simulink model "Synapse"  (Simulink 8.4)
settings: Solver=ode45  StartTime=0.0  StopTime=0.5  RelTol=1e-3
libraries: NeuroModelerLibrary x5
settings Model: Creator=Tim  LastModifiedBy=Tim
settings OptimizationCC: InitFltsAndDblsToZero=on

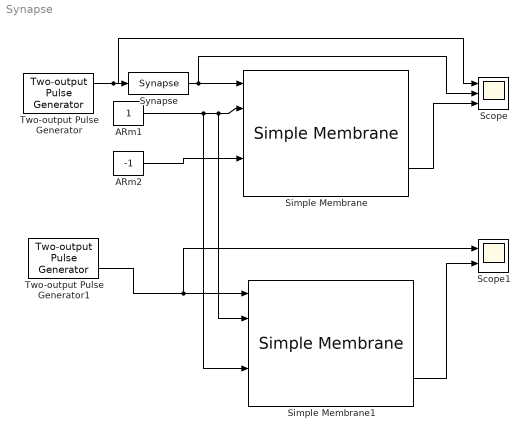
== system Synapse ==
  ARm1 : Constant
  ARm2 : Constant  Value=-1
  Scope : Scope  NumInputPorts=3
      settings: YMin=-1~0~-1  YMax=1~1e-07~0
  Scope1 : Scope  NumInputPorts=2
      settings: YMin=0~0  YMax=5e-08~1
  Simple Membrane : NeuroModelerLibrary/Neuron Elements/Simple Membrane  ACm=1e-9  ARm=1e7  ECm=1e-9  ERm=1e7  ARFm=1e8  ERFm=1e8
  Simple Membrane1 : NeuroModelerLibrary/Neuron Elements/Simple Membrane  ACm=1e-9  ARm=1e7  ECm=1e-9  ERm=1e7  ARFm=1e8  ERFm=1e8
  Synapse : NeuroModelerLibrary/Neuron Elements/Synapse  SecretionTC=0.001  DecompositionTC=0.01  ksi=2  gamma=1e7
  Two-output Pulse Generator : NeuroModelerLibrary/Support/Two-output Pulse Generator  A=1  P1=200  P2=200  PW=1  ST=0.001  OOn1=0.3  OOff1=0.6  OOn2=1.1  OOff2=1.2
  Two-output Pulse Generator1 : NeuroModelerLibrary/Support/Two-output Pulse Generator  A=5/1e8  P1=200  P2=200  PW=1  ST=1  OOn1=0.3  OOff1=0.6  OOn2=0.2  OOff2=1.2
  wires:
  ARm1/1 -> Simple Membrane/2, Simple Membrane1/2, Simple Membrane1/4
  ARm2/1 -> Simple Membrane/4
  Simple Membrane/2 -> Scope/3
  Two-output Pulse Generator/1 -> Scope/1, Synapse/1
  Synapse/1 -> Scope/2, Simple Membrane/1
  Two-output Pulse Generator1/2 -> Scope1/1, Simple Membrane1/1
  Simple Membrane1/2 -> Scope1/2
